simulink model "simulation_system"  (R2021b)
settings: Solver=VariableStepAuto  StartTime=0.0  StopTime=20  RelTol=1e-3
values from neighbouring files (symbols this model uses):
  A_I = [1 delta_t; 0 1]    [run_script.m]
  A_V = [eye(2) delta_t*eye(2) zeros(2); zeros(2) eye(2) zeros(2); zeros(2) zeros(2) zeros(2)]    [run_script.m]
  B_V = [0 0 0; 1/2*delta_t^2 0 0; 0 0 0; delta_t 0 0; 0 0 0; 1 0 0]    [run_script.m]
  beta = pi/180*45    (= 0.785398163397)    [run_script.m]
  C_I = [1 0; 0 1]    [run_script.m]
  delta_t = 0.01    [run_script.m]
  g = 9.81    [run_script.m]
  gamma = beta - atan((h_sensor-(h_box/2))/(l_sensor-(l_box/2)))    [run_script.m]
  h_box = 0.06    [run_script.m]
  h_sensor = 0.05    [run_script.m]
  l_box = 0.12    [run_script.m]
  l_sensor = 0.09    [run_script.m]
  R = sqrt((l_sensor-(l_box/2))^2 + (h_sensor-(h_box/2))^2)    [run_script.m]
  R_I = 0.01    [run_script.m]
  R_V = 0.01    [run_script.m]
  theta0 = pi/180*30    (= 0.523598775598)    [run_script.m]
  theta_v0 = pi/180*60    (= 1.0471975512)    [run_script.m]
  v0 = 100    [run_script.m]
  w0 = pi/180*180    (= 3.14159265359)    [run_script.m]
undefined symbols (not defined in the file or in its folder): Discrete, magnitude, Time
libraries: simulink x2, ctrlSharedLib x2
settings Model: PacingRate=0.010000  Creator=weera  LastModifiedBy=tatit

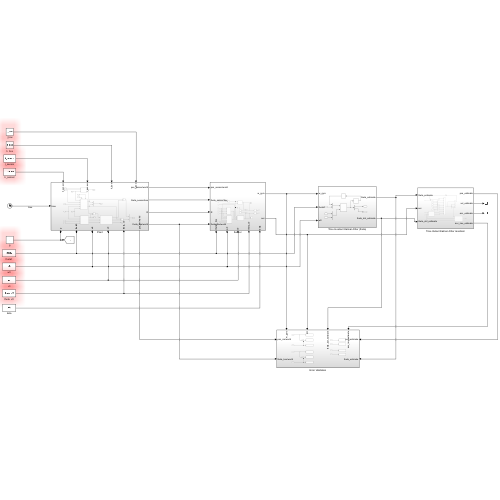
[thumbnail: Simulink's stored preview of the top-level diagram]
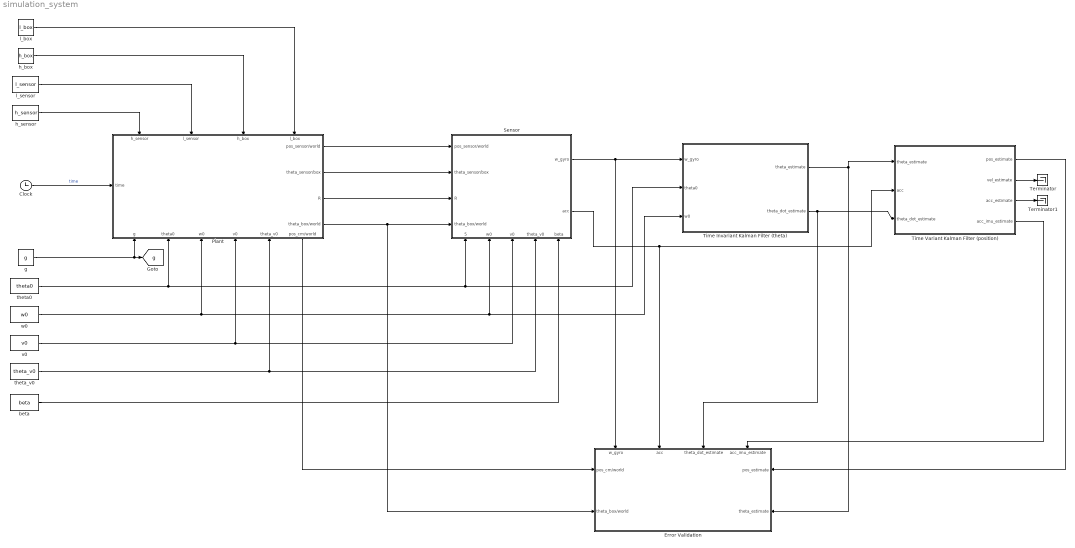
== system simulation_system ==
  Clock : Clock
  Error Validation : Subsystem
      settings: PortSchema="{\"entries\":[{\"content\":{\"sides\":[{\"content\":{\"connectorIds\":[\"In1\",\"In2\"]},\"type\":\"ConnectorPlacement.EquallySpacedRectSide\",\"uuid\":\"96552a51-5eda-48f2-b081-41a732fe48df\"},{\"content\":{\"connectorIds\":[\"In7\",\"In8\"],\"side\":\"RIGHT\"},\"type\":\"ConnectorPlacement.EquallySpacedRectSide\",\"uuid\":\"9cc494bd-ce2e-4138-b170-4221ad10e59b\"},{\"content\":{\"connectorIds\":[\"In3\",\"In4\",\"In5\",\"In6\"],\"side\":\"TOP\"},\"type\":\"ConnectorPlacement.EquallySpacedRectSide\",\"uuid\":\"1d6fc715-fb79-4b7c-a17b-0ee5669a0c4a\"}]},\"type\":\"ConnectorPlacement.EquallySpacedConnector\",\"uuid\":\"9502b703-534c-48a9-9cfa-952e8451935e\"}],\"packageUris\":[\"http://schema.mathworks.com/mf0/Connector/R2020b\"],\"version\":\"1.0\"}"
  Plant : Subsystem
      settings: PortSchema="{\"entries\":[{\"content\":{\"sides\":[{\"content\":{\"connectorIds\":[\"In1\"]},\"type\":\"ConnectorPlacement.EquallySpacedRectSide\",\"uuid\":\"b3500672-af78-425f-83aa-1ce7e56cb401\"},{\"content\":{\"connectorIds\":[\"Out1\",\"Out2\",\"Out3\",\"Out4\"],\"side\":\"RIGHT\"},\"type\":\"ConnectorPlacement.EquallySpacedRectSide\",\"uuid\":\"baf3546a-67aa-4774-be2f-5a09aa43a81d\"},{\"content\":{\"connectorIds\":[\"In2\",\"In3\",\"In4\",\"In5\"],\"side\":\"TOP\"},\"type\":\"ConnectorPlacement.EquallySpacedRectSide\",\"uuid\":\"50adaed3-2c22-42a3-879b-4acb6940e21d\"},{\"content\":{\"connectorIds\":[\"In6\",\"In7\",\"In8\",\"In9\",\"In10\",\"Out5\"],\"side\":\"BOTTOM\"},\"type\":\"ConnectorPlacement.EquallySpacedRectSide\",\"uuid\":\"949445ea-1514-4232-a9d9-9683cdf7bffb\"}]},\"type\":\"ConnectorPlacement.EquallySpacedConnector\",\"uuid\":\"04a60e30-ff30-4ae8-9de5-3960ac57b329\"}],\"packageUris\":[\"http://schema.mathworks.com/mf0/Connector/R2020b\"],\"version\":\"1.0\"}"
  Sensor : Subsystem
      settings: PortSchema="{\"entries\":[{\"content\":{\"sides\":[{\"content\":{\"connectorIds\":[\"In1\",\"In2\",\"In3\",\"In4\"]},\"type\":\"ConnectorPlacement.EquallySpacedRectSide\",\"uuid\":\"99dcf2dc-90d8-428d-bebb-7a29ab25214b\"},{\"content\":{\"connectorIds\":[\"Out1\",\"Out2\"],\"side\":\"RIGHT\"},\"type\":\"ConnectorPlacement.EquallySpacedRectSide\",\"uuid\":\"d6baf0b9-25ad-458f-bbbb-ef6e13ab1b69\"},{\"content\":{\"connectorIds\":[],\"side\":\"TOP\"},\"type\":\"ConnectorPlacement.EquallySpacedRectSide\",\"uuid\":\"34be9477-094b-465e-852f-8db332179b98\"},{\"content\":{\"connectorIds\":[\"In5\",\"In6\",\"In7\",\"In8\",\"In9\"],\"side\":\"BOTTOM\"},\"type\":\"ConnectorPlacement.EquallySpacedRectSide\",\"uuid\":\"fd6fca9d-a9e0-4c91-a866-8f96967dddac\"}]},\"type\":\"ConnectorPlacement.EquallySpacedConnector\",\"uuid\":\"600f5c00-2452-40d2-aeae-890b2a26022c\"}],\"packageUris\":[\"http://schema.mathworks.com/mf0/Connector/R2020b\"],\"version\":\"1.0\"}"
  Terminator : Terminator
  Terminator1 : Terminator
  Time Invariant Kalman Filter (theta) : Subsystem
  Time Variant Kalman Filter (position) : Subsystem
  beta : Constant  Value=beta
  g : Constant  Value=g
  h_box : Constant  Value=h_box
  h_sensor : Constant  Value=h_sensor
  l_box : Constant  Value=l_box
  l_sensor : Constant  Value=l_sensor
  theta0 : Constant  Value=theta0
  theta_v0 : Constant  Value=theta_v0
  v0 : Constant  Value=v0
  w0 : Constant  Value=w0
  tag scope: g=global
  wires:
  Clock/1 -> Plant/1(time)  "time"
  h_box/1 -> Plant/4(h_box)
  l_box/1 -> Plant/5(l_box)
  g/1 -> Plant/6(g), [g]
  theta0/1 -> Time Invariant Kalman Filter (theta)/2(theta0), Sensor/5(theta0_box), Plant/7(theta0)
  w0/1 -> Time Invariant Kalman Filter (theta)/3(w0), Sensor/6(w0), Plant/8(w0)
  v0/1 -> Sensor/7(v0), Plant/9(v0)
  theta_v0/1 -> Sensor/8(theta_v0), Plant/10(theta_v0)
  h_sensor/1 -> Plant/2(h_sensor)
  l_sensor/1 -> Plant/3(l_sensor)
  beta/1 -> Sensor/9(beta)
  Plant/1(pos_sensor/world) -> Sensor/1(pos_sensor/world)
  Plant/5(pos_cm/world) -> Error Validation/1(pos_cm/world)
  Plant/2(theta_sensor/box) -> Sensor/2(theta_sensor/box)
  Plant/3(R) -> Sensor/3(R)
  Plant/4(theta_box/world) -> Error Validation/2(theta_box/world), Sensor/4(theta_box/world)
  Sensor/1(w_gyro) -> Time Invariant Kalman Filter (theta)/1(w_gyro), Error Validation/3(w_gyro)
  Time Invariant Kalman Filter (theta)/1(theta_estimate) -> Time Variant Kalman Filter (position)/1(theta_estimate), Error Validation/8(theta_estimate)
  Sensor/2(acc) -> Time Variant Kalman Filter (position)/2(acc), Error Validation/4(acc)
  Time Invariant Kalman Filter (theta)/2(theta_dot_estimate) -> Time Variant Kalman Filter (position)/3(theta_dot_estimate), Error Validation/5(theta_dot_estimate)
  Time Variant Kalman Filter (position)/1(pos_estimate) -> Error Validation/7(pos_estimate)
  Time Variant Kalman Filter (position)/2(vel_estimate) -> Terminator/1
  Time Variant Kalman Filter (position)/3(acc_estimate) -> Terminator1/1
  Time Variant Kalman Filter (position)/4(acc_imu_estimate) -> Error Validation/6(acc_imu_estimate)

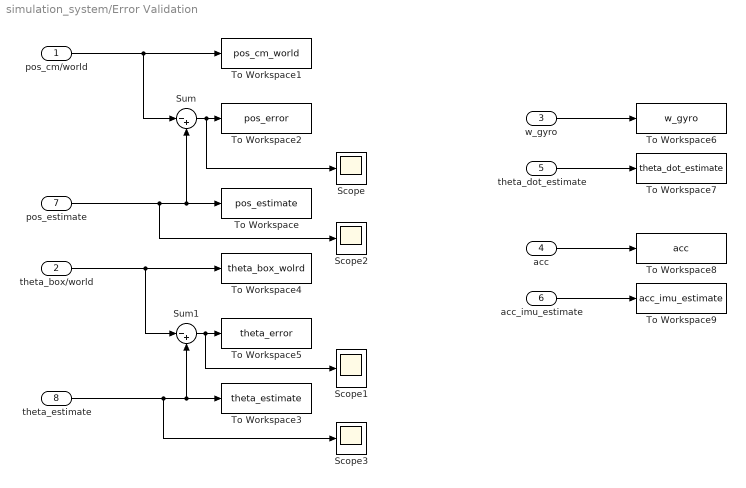
== system simulation_system/Error Validation ==
  pos_cm/world : Inport
  theta_box/world : Inport  Port=2
  w_gyro : Inport  Port=3
  acc : Inport  Port=4
  theta_dot_estimate : Inport  Port=5
  acc_imu_estimate : Inport  Port=6
  pos_estimate : Inport  Port=7
  theta_estimate : Inport  Port=8
  Scope{,1..3} (4 alike) : Scope
  Sum : Sum  Inputs=|-+
  Sum1 : Sum  Inputs=|-+
  To Workspace : ToWorkspace  VariableName=pos_estimate  SaveFormat=Timeseries  SampleTime=delta_t
  To Workspace1 : ToWorkspace  VariableName=pos_cm_world  SaveFormat=Timeseries  SampleTime=delta_t
  To Workspace2 : ToWorkspace  VariableName=pos_error  SaveFormat=Timeseries  SampleTime=delta_t
  To Workspace3 : ToWorkspace  VariableName=theta_estimate  SaveFormat=Timeseries  SampleTime=delta_t
  To Workspace4 : ToWorkspace  VariableName=theta_box_wolrd  SaveFormat=Timeseries  SampleTime=delta_t
  To Workspace5 : ToWorkspace  VariableName=theta_error  SaveFormat=Timeseries  SampleTime=delta_t
  To Workspace6 : ToWorkspace  VariableName=w_gyro  SaveFormat=Timeseries  SampleTime=delta_t
  To Workspace7 : ToWorkspace  VariableName=theta_dot_estimate  SaveFormat=Timeseries  SampleTime=delta_t
  To Workspace8 : ToWorkspace  VariableName=acc  SaveFormat=Timeseries  SampleTime=delta_t
  To Workspace9 : ToWorkspace  VariableName=acc_imu_estimate  SaveFormat=Timeseries  SampleTime=delta_t
  wires:
  pos_estimate/1 -> Scope2/1, Sum/2, To Workspace/1
  pos_cm/world/1 -> Sum/1, To Workspace1/1
  Sum/1 -> Scope/1, To Workspace2/1
  theta_box/world/1 -> Sum1/1, To Workspace4/1
  Sum1/1 -> Scope1/1, To Workspace5/1
  theta_estimate/1 -> Scope3/1, Sum1/2, To Workspace3/1
  w_gyro/1 -> To Workspace6/1
  theta_dot_estimate/1 -> To Workspace7/1
  acc/1 -> To Workspace8/1
  acc_imu_estimate/1 -> To Workspace9/1

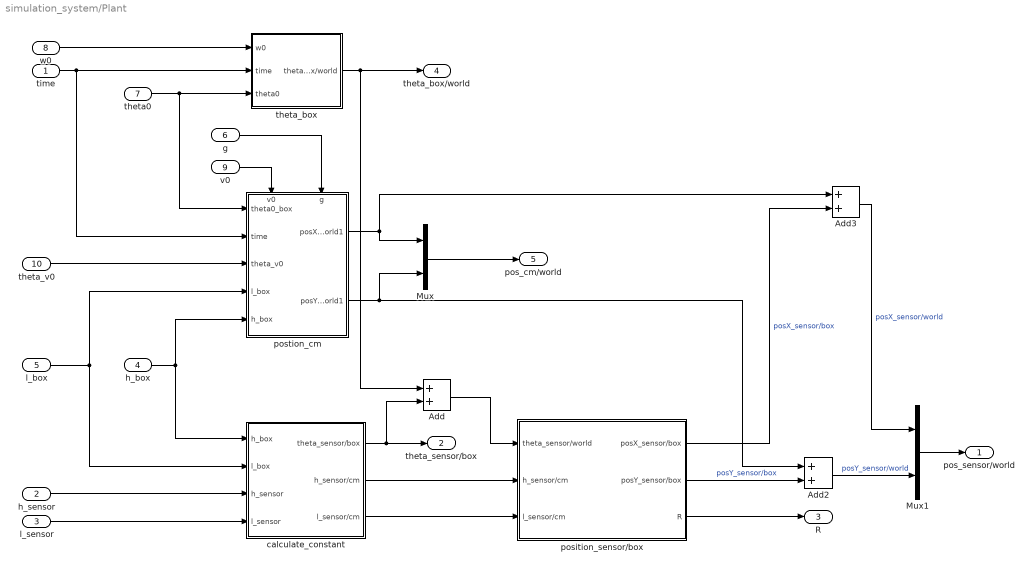
== system simulation_system/Plant ==
  time : Inport
  h_sensor : Inport  Port=2
  l_sensor : Inport  Port=3
  h_box : Inport  Port=4
  l_box : Inport  Port=5
  g : Inport  Port=6
  theta0 : Inport  Port=7
  w0 : Inport  Port=8
  v0 : Inport  Port=9
  theta_v0 : Inport  Port=10
  Add : Sum
  Add2 : Sum
  Add3 : Sum
  Mux : Mux  Inputs=2
  Mux1 : Mux  Inputs=2
  calculate_constant : Subsystem
  position_sensor/box : Subsystem
  postion_cm : Subsystem
      settings: PortSchema="{\"entries\":[{\"content\":{\"sides\":[{\"content\":{\"connectorIds\":[\"In1\",\"In2\",\"In3\",\"In4\",\"In5\"]},\"type\":\"ConnectorPlacement.EquallySpacedRectSide\",\"uuid\":\"18064696-ad63-4c6f-8f3f-5b4e0b983ed5\"},{\"content\":{\"connectorIds\":[\"Out1\",\"Out2\"],\"side\":\"RIGHT\"},\"type\":\"ConnectorPlacement.EquallySpacedRectSide\",\"uuid\":\"5ae04fe6-84a0-457a-afb8-1002c11a5862\"},{\"content\":{\"connectorIds\":[\"In6\",\"In7\"],\"side\":\"TOP\"},\"type\":\"ConnectorPlacement.EquallySpacedRectSide\",\"uuid\":\"a330c107-137b-48ce-a9ca-8f8e635d2dd0\"},{\"content\":{\"connectorIds\":[],\"side\":\"BOTTOM\"},\"type\":\"ConnectorPlacement.EquallySpacedRectSide\",\"uuid\":\"d39472f6-a6cc-4e39-8294-838b2dbe8b15\"}]},\"type\":\"ConnectorPlacement.EquallySpacedConnector\",\"uuid\":\"8a0be8d2-740e-4315-9ddd-6bae0655516f\"}],\"packageUris\":[\"http://schema.mathworks.com/mf0/Connector/R2020b\"],\"version\":\"1.0\"}"
  theta_box : Subsystem
  pos_sensor/world : Outport
  theta_sensor/box : Outport  Port=2
  R : Outport  Port=3
  theta_box/world : Outport  Port=4
  pos_cm/world : Outport  Port=5
  wires:
  h_sensor/1 -> calculate_constant/3(h_sensor)
  l_sensor/1 -> calculate_constant/4(l_sensor)
  position_sensor/box/3(R) -> R/1
  calculate_constant/2(h_sensor/cm) -> position_sensor/box/2(h_sensor/cm)
  calculate_constant/3(l_sensor/cm) -> position_sensor/box/3(l_sensor/cm)
  Add3/1 -> Mux1/1  "posX_sensor/world"
  Add2/1 -> Mux1/2  "posY_sensor/world"
  Mux/1 -> pos_cm/world/1
  position_sensor/box/1(posX_sensor/box) -> Add3/2  "posX_sensor/box"
  theta0/1 -> theta_box/3(theta0), postion_cm/1(theta0_box)
  position_sensor/box/2(posY_sensor/box) -> Add2/2  "posY_sensor/box"
  Add/1 -> position_sensor/box/1(theta_sensor/world)
  w0/1 -> theta_box/1(w0)
  Mux1/1 -> pos_sensor/world/1
  calculate_constant/1(theta_sensor/box) -> Add/2, theta_sensor/box/1
  h_box/1 -> postion_cm/5(h_box), calculate_constant/1(h_box)
  l_box/1 -> postion_cm/4(l_box), calculate_constant/2(l_box)
  theta_box/1(theta_box/world) -> theta_box/world/1, Add/1
  time/1 -> theta_box/2(time), postion_cm/2(time)
  postion_cm/1(posX_cm/world1) -> Add3/1, Mux/1
  postion_cm/2(posY_cm/world1) -> Add2/1, Mux/2
  theta_v0/1 -> postion_cm/3(theta_v0)
  v0/1 -> postion_cm/6(v0)
  g/1 -> postion_cm/7(g)

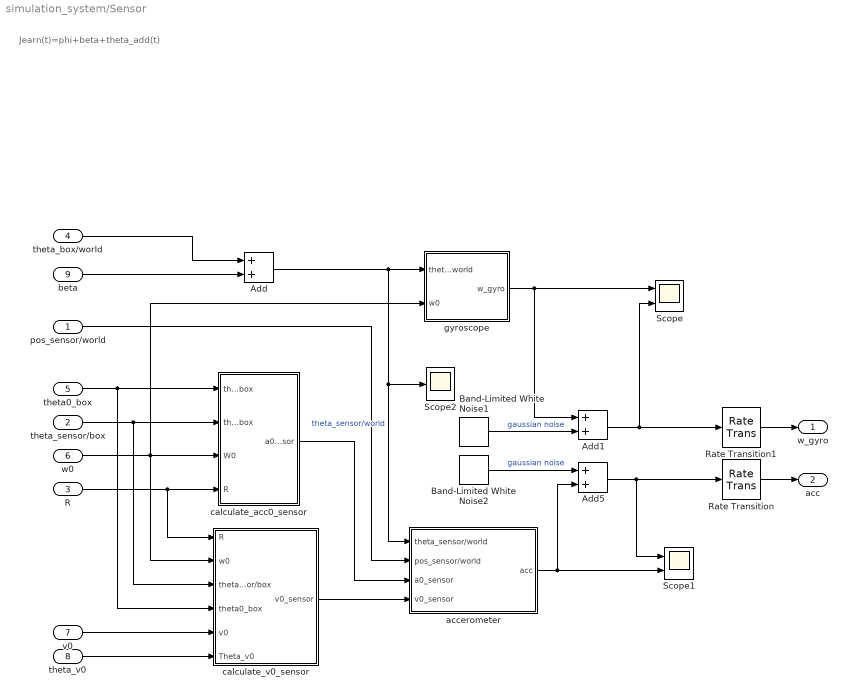
== system simulation_system/Sensor ==
  note: Jearn(t)=phi+beta+theta_add(t)
  pos_sensor/world : Inport
  theta_sensor/box : Inport  Port=2
  R : Inport  Port=3
  theta_box/world : Inport  Port=4
  theta0_box : Inport  Port=5
  w0 : Inport  Port=6
  v0 : Inport  Port=7
  theta_v0 : Inport  Port=8
  beta : Inport  Port=9
  Add : Sum
  Add1 : Sum
  Add5 : Sum
  Band-Limited White Noise1 : simulink/Sources/Band-Limited White Noise  Cov=[0.01]  Ts=0.1  seed=[23341]
  Band-Limited White Noise2 : simulink/Sources/Band-Limited White Noise  Cov=[0.01]  Ts=0.1  seed=[2331]
  Rate Transition : RateTransition  OutPortSampleTime=delta_t
  Rate Transition1 : RateTransition  OutPortSampleTime=delta_t
  Scope : Scope  NumInputPorts=2
  Scope1 : Scope  NumInputPorts=2
  Scope2 : Scope
  accerometer : Subsystem
  calculate_acc0_sensor : Subsystem
  calculate_v0_sensor : Subsystem
  gyroscope : Subsystem
  w_gyro : Outport
  acc : Outport  Port=2
  wires:
  R/1 -> calculate_acc0_sensor/4(R), calculate_v0_sensor/1(R)
  calculate_v0_sensor/1(v0_sensor) -> accerometer/4(v0_sensor)
  Rate Transition/1 -> acc/1
  Rate Transition1/1 -> w_gyro/1
  theta0_box/1 -> calculate_v0_sensor/4(theta0_box), calculate_acc0_sensor/1(theta0_box)
  v0/1 -> calculate_v0_sensor/5(v0)
  theta_v0/1 -> calculate_v0_sensor/6(Theta_v0)
  calculate_acc0_sensor/1(a0_sensor) -> accerometer/3(a0_sensor)
  theta_box/world/1 -> Add/1
  Add1/1 -> Rate Transition1/1, Scope/2
  beta/1 -> Add/2
  Band-Limited White Noise2/1 -> Add5/1  "gaussian noise"
  pos_sensor/world/1 -> accerometer/2(pos_sensor/world)
  Band-Limited White Noise1/1 -> Add1/2  "gaussian noise"
  theta_sensor/box/1 -> calculate_v0_sensor/3(theta_sensor/box), calculate_acc0_sensor/2(theta_sensor/box)
  w0/1 -> calculate_v0_sensor/2(w0), gyroscope/2(w0), calculate_acc0_sensor/3(W0)
  Add5/1 -> Scope1/1, Rate Transition/1
  Add/1 -> gyroscope/1(theta_sensor/world), Scope2/1, accerometer/1(theta_sensor/world)  "theta_sensor/world"
  accerometer/1(acc) -> Add5/2, Scope1/2
  gyroscope/1(w_gyro) -> Scope/1, Add1/1

== system simulation_system/Time Invariant Kalman Filter (theta) ==
  w_gyro : Inport
  theta0 : Inport  Port=2
  w0 : Inport  Port=3
  Demux : Demux  Outputs=2
  Kalman Filter2 : ctrlSharedLib/Kalman Filter  TimeDomain=Discrete-Time  UseCurrentEstimator=on  ModelSource=Individual A, B, C, D matrices  ModelSourceVariable=ss(0.95,1,1,0,1)  A=A_I  B=1  C=C_I  D=0  NumberOfStates=1  NumberOfInputs=1  NumberOfOutputs=1  InitialEstimateSource=Input port  X0=[0 2]  P0=10  UseK=off  UseGH=on  NumberOfProcessNoiseInputs=1  G=G_I  TimeInvariantG=on  H=H_I  TimeInvariantH=on  Q=Q_I  TimeInvariantQ=on  R=R_I  TimeInvariantR=on  N=0  TimeInvariantN=on  AddInputPort=off  AddEnablePort=off  OutputEstimatedY=off  OutputP=off  Ts=delta_t
  Mux : Mux  Inputs=2
  Mux1 : Mux  Inputs=2
  Selector2 : Selector  InputPortWidth=2  IndexOptions=Index vector (dialog)  Indices=[1]  OutputSizes=1
  Unit Delay : UnitDelay  SampleTime=delta_t  HasFrameUpgradeWarning=on
  theta_estimate : Outport
  theta_dot_estimate : Outport  Port=2
  wires:
  theta0/1 -> Mux/1
  w0/1 -> Mux/2
  Demux/1 -> theta_estimate/1
  Demux/2 -> theta_dot_estimate/1
  Selector2/1 -> Unit Delay/1
  Kalman Filter2/1 -> Demux/1, Selector2/1
  Mux1/1 -> Kalman Filter2/1
  w_gyro/1 -> Mux1/2
  Mux/1 -> Kalman Filter2/2
  Unit Delay/1 -> Mux1/1

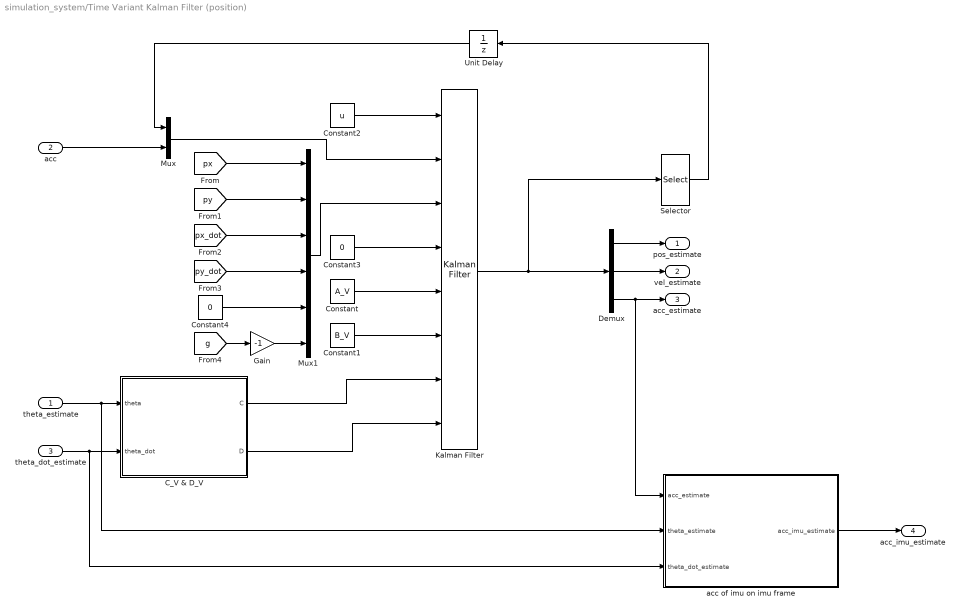
== system simulation_system/Time Variant Kalman Filter (position) ==
  theta_estimate : Inport
  acc : Inport  Port=2
  theta_dot_estimate : Inport  Port=3
  C_V & D_V : Subsystem
  Constant : Constant  Value=A_V  SampleTime=delta_t
  Constant1 : Constant  Value=B_V  SampleTime=delta_t
  Constant2 : Constant  Value=u  SampleTime=delta_t
  Constant3 : Constant  Value=0
  Constant4 : Constant  Value=0  SampleTime=delta_t
  Demux : Demux  Outputs=3
  Gain : Gain  Gain=-1
  Kalman Filter : ctrlSharedLib/Kalman Filter  TimeDomain=Discrete-Time  UseCurrentEstimator=on  ModelSource=Input port  ModelSourceVariable=ss(0.95,1,1,0,1)  A=0.95  B=1  C=1  D=0  NumberOfStates=6  NumberOfInputs=3  NumberOfOutputs=6  InitialEstimateSource=Input port  X0=0  P0=10  UseK=off  UseGH=on  NumberOfProcessNoiseInputs=1  G=G_V  TimeInvariantG=on  H=H_V  TimeInvariantH=on  Q=Q_V  TimeInvariantQ=on  R=R_V  TimeInvariantR=on  N=0  TimeInvariantN=on  AddInputPort=on  AddEnablePort=off  OutputEstimatedY=off  OutputP=off  Ts=delta_t
  Mux : Mux  Inputs=2
  Mux1 : Mux  Inputs=6
  Selector : Selector  InputPortWidth=6  IndexOptions=Index vector (dialog)  Indices=[1 2 3 4]  OutputSizes=1
  Unit Delay : UnitDelay  SampleTime=-1  HasFrameUpgradeWarning=on
  acc of imu on imu frame : Subsystem
  pos_estimate : Outport
  vel_estimate : Outport  Port=2
  acc_estimate : Outport  Port=3
  acc_imu_estimate : Outport  Port=4
  wires:
  [px] -> Mux1/1
  Constant3/1 -> Kalman Filter/4
  [py_dot] -> Mux1/4
  Mux1/1 -> Kalman Filter/3
  [g] -> Gain/1
  Kalman Filter/1 -> Selector/1, Demux/1
  acc/1 -> Mux/2
  Gain/1 -> Mux1/6
  Selector/1 -> Unit Delay/1
  Unit Delay/1 -> Mux/1
  [py] -> Mux1/2
  Constant1/1 -> Kalman Filter/6
  Constant/1 -> Kalman Filter/5
  Mux/1 -> Kalman Filter/2
  Constant2/1 -> Kalman Filter/1
  C_V & D_V/2(D) -> Kalman Filter/8
  C_V & D_V/1(C) -> Kalman Filter/7
  [px_dot] -> Mux1/3
  Constant4/1 -> Mux1/5
  theta_estimate/1 -> acc of imu on imu frame/2(theta_estimate), C_V & D_V/1(theta)
  Demux/1 -> pos_estimate/1
  Demux/2 -> vel_estimate/1
  Demux/3 -> acc of imu on imu frame/1(acc_estimate), acc_estimate/1
  acc of imu on imu frame/1(acc_imu_estimate) -> acc_imu_estimate/1
  theta_dot_estimate/1 -> C_V & D_V/2(theta_dot), acc of imu on imu frame/3(theta_dot_estimate)

== system simulation_system/Plant/calculate_constant ==
  h_box : Inport
  l_box : Inport  Port=2
  h_sensor : Inport  Port=3
  l_sensor : Inport  Port=4
  Divide : Product  Inputs=*/
  Gain2 : Gain  Gain=0.5
  Gain3 : Gain  Gain=0.5
  Subtract : Sum  Inputs=+-
  Subtract1 : Sum  Inputs=+-
  Tan : Trigonometry  Operator=atan
  theta_sensor/box : Outport
  h_sensor/cm : Outport  Port=2
  l_sensor/cm : Outport  Port=3
  wires:
  Subtract1/1 -> Divide/1, h_sensor/cm/1
  h_box/1 -> Gain2/1
  h_sensor/1 -> Subtract1/1
  Subtract/1 -> l_sensor/cm/1, Divide/2  "L_sensor/cm"
  Gain2/1 -> Subtract1/2
  Gain3/1 -> Subtract/2
  Tan/1 -> theta_sensor/box/1
  Divide/1 -> Tan/1
  l_sensor/1 -> Subtract/1
  l_box/1 -> Gain3/1

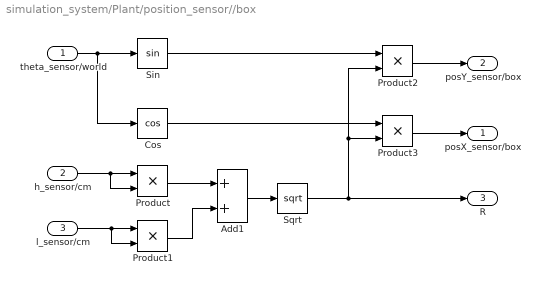
== system simulation_system/Plant/position_sensor//box ==
  theta_sensor/world : Inport
  h_sensor/cm : Inport  Port=2
  l_sensor/cm : Inport  Port=3
  Add1 : Sum
  Cos : Trigonometry  Operator=cos
  Product{,1..3} (4 alike) : Product
  Sin : Trigonometry
  Sqrt : Sqrt  SaturateOnIntegerOverflow=on
  posX_sensor/box : Outport
  posY_sensor/box : Outport  Port=2
  R : Outport  Port=3
  wires:
  theta_sensor/world/1 -> Cos/1, Sin/1
  Product2/1 -> posY_sensor/box/1
  Cos/1 -> Product3/1
  Sin/1 -> Product2/1
  Product3/1 -> posX_sensor/box/1
  Sqrt/1 -> Product2/2, Product3/2, R/1
  Add1/1 -> Sqrt/1
  Product/1 -> Add1/1
  Product1/1 -> Add1/2
  h_sensor/cm/1 -> Product/2, Product/1
  l_sensor/cm/1 -> Product1/2, Product1/1

== system simulation_system/Plant/postion_cm ==
  theta0_box : Inport
  time : Inport  Port=2
  theta_v0 : Inport  Port=3
  l_box : Inport  Port=4
  h_box : Inport  Port=5
  v0 : Inport  Port=6
  g : Inport  Port=7
  posX_cm/world : Subsystem
  posY_cm/world : Subsystem
  posX_cm/world1 : Outport
  posY_cm/world1 : Outport  Port=2
  wires:
  theta0_box/1 -> posX_cm/world/2(theta0_box), posY_cm/world/6(theta0_box)
  theta_v0/1 -> posY_cm/world/2(theta_v), posX_cm/world/3(theta_v)
  posX_cm/world/1(posX_cm/world2) -> posX_cm/world1/1
  posY_cm/world/1(posY_cm/world) -> posY_cm/world1/1
  v0/1 -> posY_cm/world/1(v0), posX_cm/world/6(v0)
  time/1 -> posY_cm/world/3(time), posX_cm/world/1(time)
  h_box/1 -> posY_cm/world/5(h_box), posX_cm/world/5(h_box)
  g/1 -> posY_cm/world/7(g)
  l_box/1 -> posY_cm/world/4(l_box), posX_cm/world/4(l_box)

== system simulation_system/Plant/theta_box ==
  w0 : Inport
  time : Inport  Port=2
  theta0 : Inport  Port=3
  Add : Sum
  Product : Product
  theta_box/world : Outport
  wires:
  w0/1 -> Product/1
  Product/1 -> Add/1
  Add/1 -> theta_box/world/1
  theta0/1 -> Add/2
  time/1 -> Product/2

== system simulation_system/Sensor/accerometer ==
  theta_sensor/world : Inport
  pos_sensor/world : Inport  Port=2
  a0_sensor : Inport  Port=3
  v0_sensor : Inport  Port=4
  Clock : Clock
  P_to acc_world : Subsystem
  transform axis : Subsystem
  acc : Outport
  wires:
  theta_sensor/world/1 -> transform axis/1(theta_sensor/world)
  transform axis/1(acc) -> acc/1
  pos_sensor/world/1 -> P_to acc_world/1(pos_sensor/world)
  v0_sensor/1 -> P_to acc_world/2(v0_sensor)
  Clock/1 -> P_to acc_world/3(t)
  a0_sensor/1 -> P_to acc_world/4(a0_sensor)
  P_to acc_world/1(accX_sensor/world) -> transform axis/2(accX_sensor/world)
  P_to acc_world/2(accY_sensor/world) -> transform axis/3(accY_sensor/world)

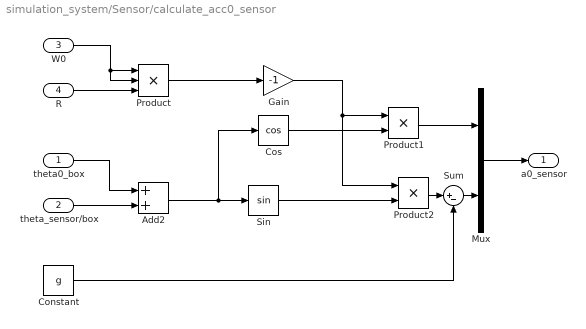
== system simulation_system/Sensor/calculate_acc0_sensor ==
  theta0_box : Inport
  theta_sensor/box : Inport  Port=2
  W0 : Inport  Port=3
  R : Inport  Port=4
  Add2 : Sum
  Constant : Constant  Value=g
  Cos : Trigonometry  Operator=cos
  Gain : Gain  Gain=-1
  Mux : Mux  Inputs=2
  Product : Product  Inputs=3
  Product1 : Product
  Product2 : Product
  Sin : Trigonometry
  Sum : Sum  Inputs=|+-
  a0_sensor : Outport
  wires:
  Sin/1 -> Product2/2
  Product/1 -> Gain/1
  W0/1 -> Product/2, Product/1
  Gain/1 -> Product1/1, Product2/1
  Product1/1 -> Mux/1
  theta_sensor/box/1 -> Add2/2
  Add2/1 -> Cos/1, Sin/1
  R/1 -> Product/3
  Cos/1 -> Product1/2
  Mux/1 -> a0_sensor/1
  theta0_box/1 -> Add2/1
  Constant/1 -> Sum/2
  Product2/1 -> Sum/1
  Sum/1 -> Mux/2

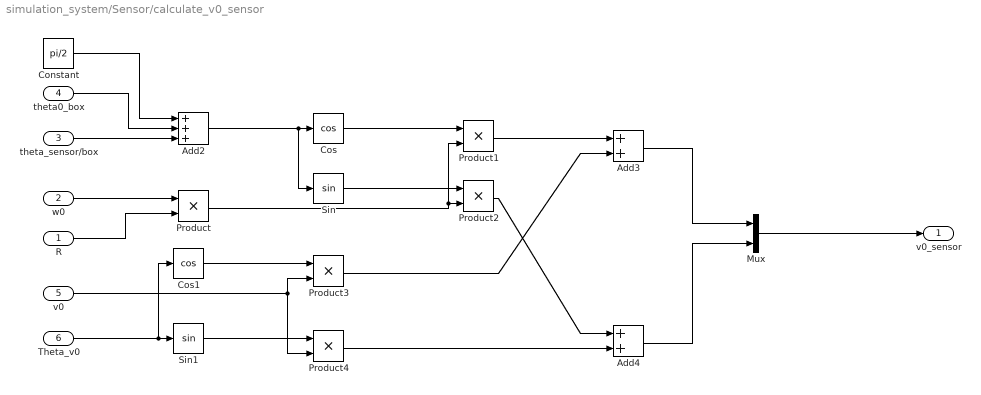
== system simulation_system/Sensor/calculate_v0_sensor ==
  R : Inport
  w0 : Inport  Port=2
  theta_sensor/box : Inport  Port=3
  theta0_box : Inport  Port=4
  v0 : Inport  Port=5
  Theta_v0 : Inport  Port=6
  Add2 : Sum  Inputs=+++
  Add3 : Sum
  Add4 : Sum
  Constant : Constant  Value=pi/2
  Cos : Trigonometry  Operator=cos
  Cos1 : Trigonometry  Operator=cos
  Mux : Mux  Inputs=2
  Product{,1..4} (5 alike) : Product
  Sin : Trigonometry
  Sin1 : Trigonometry
  v0_sensor : Outport
  wires:
  Sin/1 -> Product2/1
  Cos1/1 -> Product3/1
  Product1/1 -> Add3/1
  Add3/1 -> Mux/1
  Add2/1 -> Sin/1, Cos/1
  Mux/1 -> v0_sensor/1
  w0/1 -> Product/1
  Product/1 -> Product1/2, Product2/2
  theta_sensor/box/1 -> Add2/3
  Constant/1 -> Add2/1
  Product3/1 -> Add3/2
  Sin1/1 -> Product4/1
  v0/1 -> Product3/2, Product4/2
  Theta_v0/1 -> Cos1/1, Sin1/1
  Cos/1 -> Product1/1
  theta0_box/1 -> Add2/2
  R/1 -> Product/2
  Product2/1 -> Add4/1
  Product4/1 -> Add4/2
  Add4/1 -> Mux/2

== system simulation_system/Sensor/gyroscope ==
  theta_sensor/world : Inport
  w0 : Inport  Port=2
  Clock : Clock
  Derivative : Derivative
  Function w : MATLAB Function  TreatAsAtomicUnit=on
  w_gyro : Outport
  wires:
  Derivative/1 -> Function w/1(w)
  theta_sensor/world/1 -> Derivative/1
  Function w/1(w_fill) -> w_gyro/1
  Clock/1 -> Function w/3(t)
  w0/1 -> Function w/2(w0)

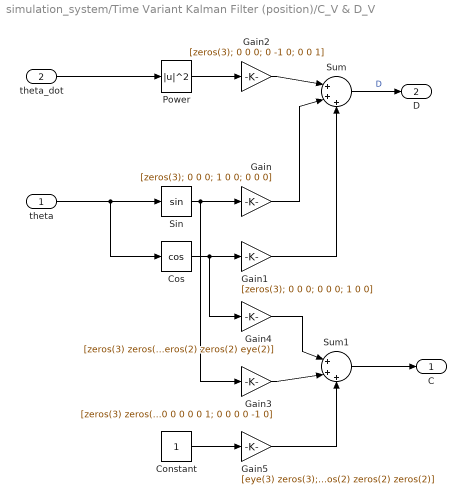
== system simulation_system/Time Variant Kalman Filter (position)/C_V & D_V ==
  theta : Inport
  theta_dot : Inport  Port=2
  Constant : Constant
  Cos : Trigonometry  Operator=cos
  Gain : Gain  Gain=[zeros(3); 0 0 0; 1 0 0; 0 0 0]
  Gain1 : Gain  Gain=[zeros(3); 0 0 0; 0 0 0; 1 0 0]
  Gain2 : Gain  Gain=[zeros(3); 0 0 0; 0 -1 0; 0 0 1]
  Gain3 : Gain  Gain=[zeros(3) zeros(3); 0 0 0 0 0 0 ; 0 0 0 0 0 1; 0 0 0 0 -1 0]
  Gain4 : Gain  Gain=[zeros(3) zeros(3); 0 0 0 0 0 0 ; zeros(2) zeros(2) eye(2)]
  Gain5 : Gain  Gain=[eye(3) zeros(3); 0 0 0 1 0 0 ; zeros(2) zeros(2) zeros(2)]
  Power : Math  Operator=magnitude^2  SaturateOnIntegerOverflow=on
  Sin : Trigonometry
  Sum : Sum  Inputs=|+++
  Sum1 : Sum  Inputs=|+++
  C : Outport
  D : Outport  Port=2
  wires:
  theta/1 -> Cos/1, Sin/1
  Power/1 -> Gain2/1
  Cos/1 -> Gain4/1, Gain1/1
  Sin/1 -> Gain/1, Gain3/1
  Sum/1 -> D/1  "D"
  theta_dot/1 -> Power/1
  Gain2/1 -> Sum/1
  Gain/1 -> Sum/2
  Gain1/1 -> Sum/3
  Constant/1 -> Gain5/1
  Gain4/1 -> Sum1/1
  Gain3/1 -> Sum1/2
  Gain5/1 -> Sum1/3
  Sum1/1 -> C/1

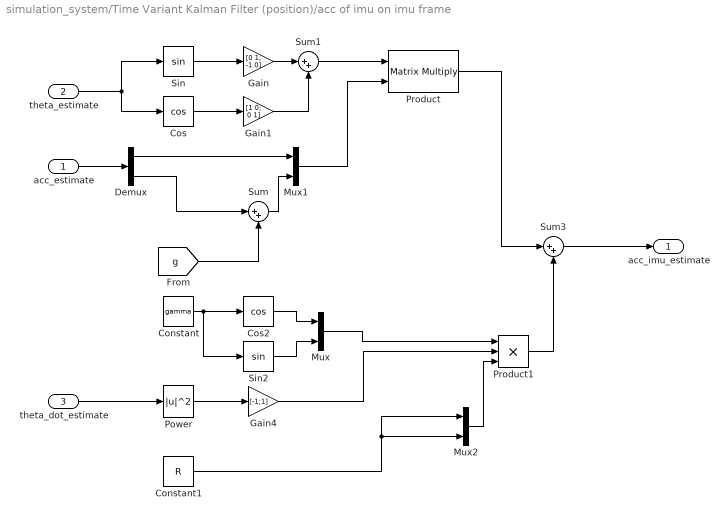
== system simulation_system/Time Variant Kalman Filter (position)/acc of imu on imu frame ==
  acc_estimate : Inport
  theta_estimate : Inport  Port=2
  theta_dot_estimate : Inport  Port=3
  Constant : Constant  Value=gamma  SampleTime=delta_t
  Constant1 : Constant  Value=R
  Cos : Trigonometry  Operator=cos
  Cos2 : Trigonometry  Operator=cos
  Demux : Demux  Outputs=2
  Gain : Gain  Gain=[0 1; -1 0]
  Gain1 : Gain  Gain=[1 0; 0 1]
  Gain4 : Gain  Gain=[-1;1]
  Mux : Mux  Inputs=2
  Mux1 : Mux  Inputs=2
  Mux2 : Mux  Inputs=2
  Power : Math  Operator=magnitude^2  SaturateOnIntegerOverflow=on
  Product : Product  Multiplication=Matrix(*)
  Product1 : Product  Inputs=3
  Sin : Trigonometry
  Sin2 : Trigonometry
  Sum : Sum  Inputs=|++
  Sum1 : Sum  Inputs=|++
  Sum3 : Sum  Inputs=|++
  acc_imu_estimate : Outport
  wires:
  Gain/1 -> Sum1/1
  Gain1/1 -> Sum1/2
  theta_estimate/1 -> Sin/1, Cos/1
  Sin/1 -> Gain/1
  Cos/1 -> Gain1/1
  Product1/1 -> Sum3/2
  Product/1 -> Sum3/1
  theta_dot_estimate/1 -> Power/1
  Sum/1 -> Mux1/2
  Power/1 -> Gain4/1
  [g] -> Sum/2
  Demux/1 -> Mux1/1
  acc_estimate/1 -> Demux/1
  Constant/1 -> Sin2/1, Cos2/1
  Demux/2 -> Sum/1
  Sum1/1 -> Product/1
  Sum3/1 -> acc_imu_estimate/1
  Cos2/1 -> Mux/1
  Sin2/1 -> Mux/2
  Mux/1 -> Product1/1
  Gain4/1 -> Product1/2
  Constant1/1 -> Mux2/2, Mux2/1
  Mux1/1 -> Product/2
  Mux2/1 -> Product1/3

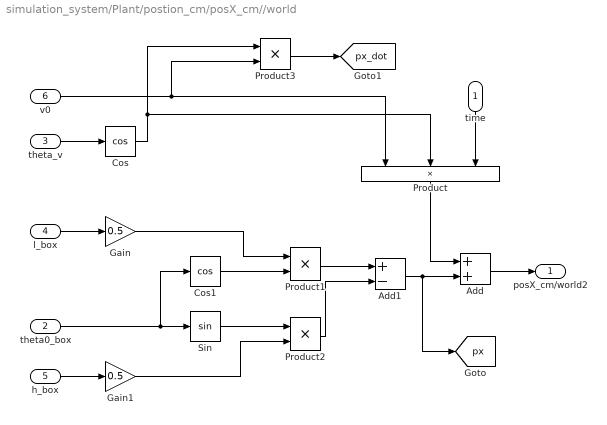
== system simulation_system/Plant/postion_cm/posX_cm//world ==
  time : Inport
  theta0_box : Inport  Port=2
  theta_v : Inport  Port=3
  l_box : Inport  Port=4
  h_box : Inport  Port=5
  v0 : Inport  Port=6
  Add : Sum
  Add1 : Sum  Inputs=+-
  Cos : Trigonometry  Operator=cos
  Cos1 : Trigonometry  Operator=cos
  Gain : Gain  Gain=0.5
  Gain1 : Gain  Gain=0.5
  Product : Product  Inputs=3
  Product1 : Product
  Product2 : Product
  Product3 : Product
  Sin : Trigonometry
  posX_cm/world2 : Outport
  tag scope: px=global, px_dot=global
  wires:
  Cos/1 -> Product3/1, Product/2
  Add/1 -> posX_cm/world2/1
  v0/1 -> Product3/2, Product/1
  Product/1 -> Add/1
  l_box/1 -> Gain/1
  theta_v/1 -> Cos/1
  time/1 -> Product/3
  h_box/1 -> Gain1/1
  theta0_box/1 -> Cos1/1, Sin/1
  Cos1/1 -> Product1/2
  Gain/1 -> Product1/1
  Product1/1 -> Add1/1
  Sin/1 -> Product2/1
  Gain1/1 -> Product2/2
  Product2/1 -> Add1/2
  Add1/1 -> [px], Add/2
  Product3/1 -> [px_dot]

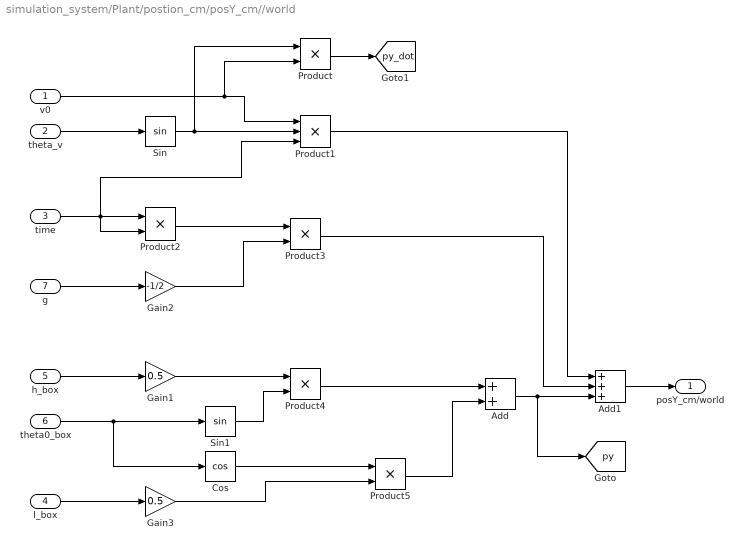
== system simulation_system/Plant/postion_cm/posY_cm//world ==
  v0 : Inport
  theta_v : Inport  Port=2
  time : Inport  Port=3
  l_box : Inport  Port=4
  h_box : Inport  Port=5
  theta0_box : Inport  Port=6
  g : Inport  Port=7
  Add : Sum
  Add1 : Sum  Inputs=+++
  Cos : Trigonometry  Operator=cos
  Gain1 : Gain  Gain=0.5
  Gain2 : Gain  Gain=-1/2
  Gain3 : Gain  Gain=0.5
  Product{,2..5} (5 alike) : Product
  Product1 : Product  Inputs=3
  Sin : Trigonometry
  Sin1 : Trigonometry
  posY_cm/world : Outport
  tag scope: py=global, py_dot=global
  wires:
  Sin/1 -> Product/1, Product1/2
  Product2/1 -> Product3/1
  time/1 -> Product2/2, Product1/3, Product2/1
  Product3/1 -> Add1/2
  h_box/1 -> Gain1/1
  v0/1 -> Product/2, Product1/1
  Gain2/1 -> Product3/2
  Product1/1 -> Add1/1
  Add1/1 -> posY_cm/world/1
  g/1 -> Gain2/1
  theta_v/1 -> Sin/1
  l_box/1 -> Gain3/1
  theta0_box/1 -> Sin1/1, Cos/1
  Gain1/1 -> Product4/1
  Sin1/1 -> Product4/2
  Product5/1 -> Add/2
  Product4/1 -> Add/1
  Cos/1 -> Product5/1
  Gain3/1 -> Product5/2
  Add/1 -> [py], Add1/3
  Product/1 -> [py_dot]

== system simulation_system/Sensor/accerometer/P_to acc_world ==
  pos_sensor/world : Inport
  v0_sensor : Inport  Port=2
  t : Inport  Port=3
  a0_sensor : Inport  Port=4
  Constant : Constant  Value=-9.81
  Demux2 : Demux  Outputs=2
  Derivative : Derivative
  Derivative2 : Derivative
  Function A : MATLAB Function  TreatAsAtomicUnit=on
  Function V : MATLAB Function  TreatAsAtomicUnit=on
  Scope : Scope  NumInputPorts=3
  Subtract : Sum  Inputs=+-
  accX_sensor/world : Outport
  accY_sensor/world : Outport  Port=2
  wires:
  Demux2/2 -> Subtract/1
  Derivative2/1 -> Function A/1(A)  "acc_sensor/world"
  pos_sensor/world/1 -> Derivative/1, Scope/3
  Derivative/1 -> Function V/1(V)  "v_sensor/world"
  Constant/1 -> Subtract/2
  Function V/1(V_fill) -> Scope/2, Derivative2/1
  t/1 -> Function V/3(t), Function A/3(t)
  a0_sensor/1 -> Function A/2(A0)
  v0_sensor/1 -> Function V/2(V0)
  Subtract/1 -> accY_sensor/world/1
  Function A/1(A_fil) -> Demux2/1, Scope/1
  Demux2/1 -> accX_sensor/world/1

== system simulation_system/Sensor/accerometer/transform axis ==
  theta_sensor/world : Inport
  accX_sensor/world : Inport  Port=2
  accY_sensor/world : Inport  Port=3
  Add1 : Sum  Inputs=-+
  Add2 : Sum
  Cos : Trigonometry  Operator=cos
  Gain : Gain  Gain=-1
  Mux : Mux  Inputs=2
  Product{,1..3} (4 alike) : Product
  Sin : Trigonometry
  acc : Outport
  wires:
  Sin/1 -> Product1/2, Product2/2
  accX_sensor/world/1 -> Product2/1, Product/2
  theta_sensor/world/1 -> Gain/1
  Product2/1 -> Add2/1
  Gain/1 -> Cos/1, Sin/1
  Add2/1 -> Mux/2
  Product1/1 -> Add1/1
  Product/1 -> Add1/2
  Product3/1 -> Add2/2
  Cos/1 -> Product3/1, Product/1
  Add1/1 -> Mux/1
  Mux/1 -> acc/1
  accY_sensor/world/1 -> Product3/2, Product1/1

== matlab function simulation_system/Sensor/accerometer/P_to acc_world/Function A ==
  data: A input; A_fil output; A0 input; t input
function A_fil = test(A,A0,t)
if t==0
    A_fil=A0;
else
    A_fil=A;
end

== matlab function simulation_system/Sensor/gyroscope/Function w ==
  data: w input; w_fill output; w0 input; t input
function w_fill = fillter_w(w,w0,t)
if t==0
    w_fill=w0;
else
    w_fill=w;
end

== matlab function simulation_system/Sensor/accerometer/P_to acc_world/Function V ==
  data: V input; V_fill output; V0 input; t input
function V_fill = fillterv(V,V0,t)
if t==0
    V_fill=V0;
else
    V_fill=V;
end
